simulink model "Ejemplo_2_Dead_Reckoning"  (R2022a)
settings: Solver=VariableStepAuto  StartTime=0.0  StopTime=10  RelTol=1e-3
undefined symbols (not defined in the file or in its folder): ticksPerRot, wheelR
libraries: simulink x2
settings Model: Creator=L03107259  LastModifiedBy=L03107259

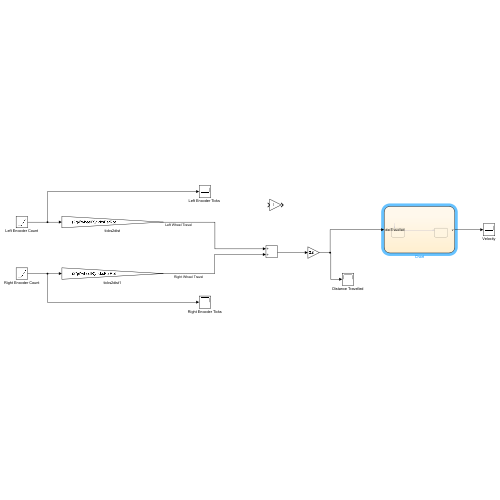
[thumbnail: Simulink's stored preview of the top-level diagram]
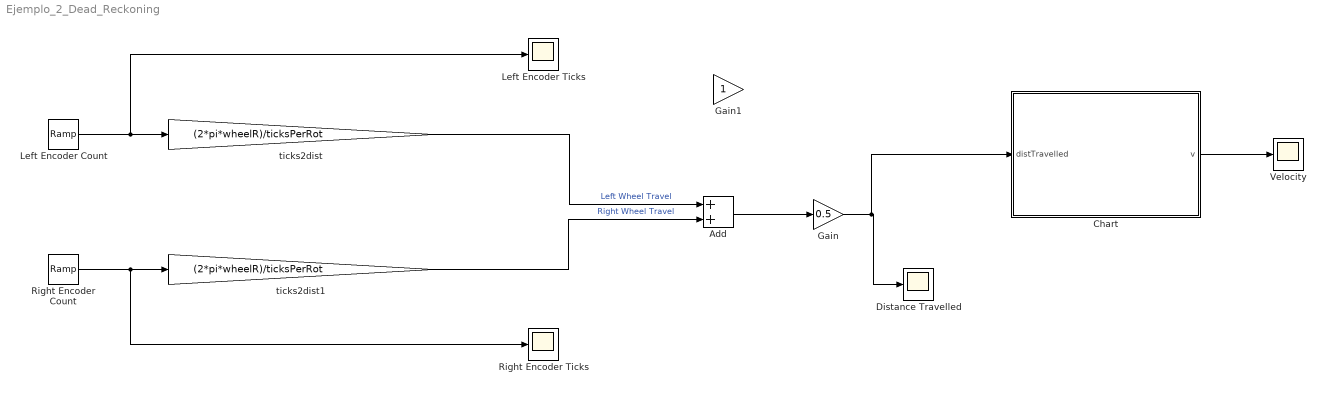
== system Ejemplo_2_Dead_Reckoning ==
  Add : Sum
  Chart : Stateflow chart  TreatAsAtomicUnit=on
  Distance Travelled : Scope
  Gain : Gain  Gain=0.5
  Gain1 : Gain
  Left Encoder Count : simulink/Sources/Ramp  slope=1  start=0  InitialOutput=0
  "Left Encoder Ticks " : Scope
  Right Encoder Count : simulink/Sources/Ramp  slope=1  start=0  InitialOutput=0
  Right Encoder Ticks : Scope
  Velocity : Scope
  ticks2dist : Gain  Gain=(2*pi*wheelR)/ticksPerRot
  ticks2dist1 : Gain  Gain=(2*pi*wheelR)/ticksPerRot
  wires:
  Left Encoder Count/1 -> "Left Encoder Ticks "/1, ticks2dist/1
  ticks2dist/1 -> Add/1  "Left Wheel Travel"
  ticks2dist1/1 -> Add/2  "Right Wheel Travel"
  Right Encoder Count/1 -> Right Encoder Ticks/1, ticks2dist1/1
  Add/1 -> Gain/1
  Gain/1 -> Chart/1(distTravelled), Distance Travelled/1
  Chart/1(v) -> Velocity/1

== stateflow chart Ejemplo_2_Dead_Reckoning/Chart ==
  state MoveForward
    entry: v=0.1;
  state Stop
    entry: v=0;
  (default) -> MoveForward : % Start
  MoveForward -> Stop : [distTravelled>=1]
  data: distTravelled input; v output
